simulink model "q11"  (R2019a)
settings: Solver=VariableStepAuto  StartTime=0.0  StopTime=0.2  RelTol=1e-3
settings Model: Creator=ADMIN  LastModifiedBy=ADMIN

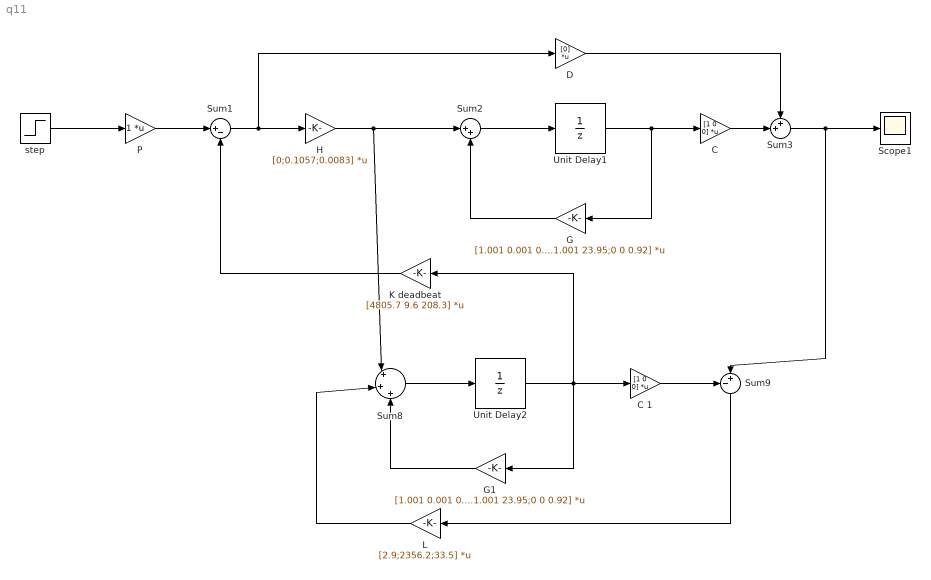
== system q11 ==
  "C " : Gain  Gain=[1 0 0]  Multiplication=Matrix(K*u)
  C 1 : Gain  Gain=[1 0 0]  Multiplication=Matrix(K*u)
  D : Gain  Gain=[0]  Multiplication=Matrix(K*u)
  G : Gain  Gain=[1.001 0.001 0.012; 1.9 1.001 23.95;0 0 0.92]  Multiplication=Matrix(K*u)
  G1 : Gain  Gain=[1.001 0.001 0.012; 1.9 1.001 23.95;0 0 0.92]  Multiplication=Matrix(K*u)
  H : Gain  Gain=[0;0.1057;0.0083]  Multiplication=Matrix(K*u)
  K deadbeat : Gain  Gain=[4805.7 9.6 208.3]  Multiplication=Matrix(K*u)
  L : Gain  Gain=[2.9;2356.2;33.5]  Multiplication=Matrix(K*u)
  P : Gain  Multiplication=Matrix(K*u)
  Scope1 : Scope
  Sum1 : Sum  Inputs=|+-
  Sum2 : Sum  Inputs=|++
  Sum3 : Sum  Inputs=++|
  Sum8 : Sum  Inputs=|+|+|+
  Sum9 : Sum  Inputs=-+|
  Unit Delay1 : UnitDelay  SampleTime=0.001  HasFrameUpgradeWarning=on
  Unit Delay2 : UnitDelay  SampleTime=0.001  HasFrameUpgradeWarning=on
  step : Step  Time=0  SampleTime=0.001
  wires:
  H/1 -> Sum2/1, Sum8/1
  Sum3/1 -> Sum9/2, Scope1/1
  Sum2/1 -> Unit Delay1/1
  D/1 -> Sum3/1
  G/1 -> Sum2/2
  Unit Delay1/1 -> G/1, "C "/1
  Sum1/1 -> H/1, D/1
  "C "/1 -> Sum3/2
  P/1 -> Sum1/1
  step/1 -> P/1
  K deadbeat/1 -> Sum1/2
  Sum8/1 -> Unit Delay2/1
  Unit Delay2/1 -> G1/1, K deadbeat/1, C 1/1
  C 1/1 -> Sum9/1
  Sum9/1 -> L/1
  L/1 -> Sum8/2
  G1/1 -> Sum8/3
